simulink model "velocityInRadiusOut"  (R2019a)
settings: Solver=VariableStepAuto  StartTime=0  StopTime=init.maxV  MaxStep=1e-3  RelTol=1e-3
undefined symbols (not defined in the file or in its folder): init
libraries: simulink x1
settings Model: Creator=fried  LastModifiedBy=fried

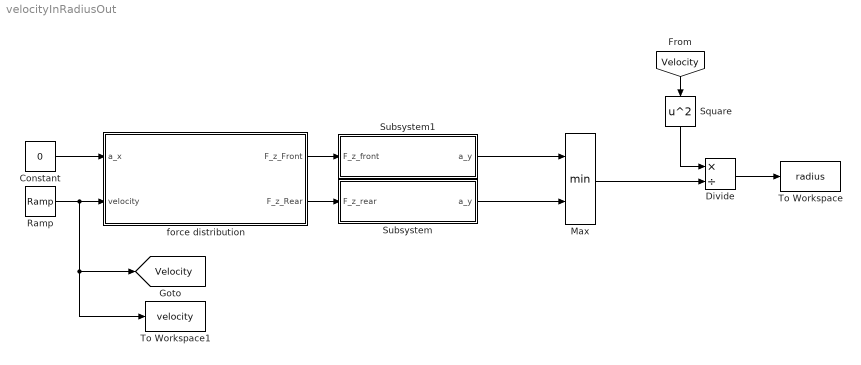
== system velocityInRadiusOut ==
  Constant : Constant  Value=0
  Divide : Product  Inputs=*/
  Max : MinMax  Inputs=2
  Ramp : simulink/Sources/Ramp  slope=1  start=0  InitialOutput=0
  Square : Math  Operator=square  SaturateOnIntegerOverflow=on
  Subsystem : Subsystem
  Subsystem1 : Subsystem
  To Workspace : ToWorkspace  VariableName=radius  SampleTime=-1
  To Workspace1 : ToWorkspace  VariableName=velocity  SampleTime=-1
  force distribution : Subsystem
  tag scope: Velocity=global
  wires:
  Ramp/1 -> To Workspace1/1, [Velocity], force distribution/2("velocity ")
  force distribution/2("F_z_Rear ") -> Subsystem/1("F_z_rear ")
  force distribution/1(F_z_Front) -> Subsystem1/1(F_z_front)
  Subsystem1/1(a_y) -> Max/1
  [Velocity] -> Square/1
  Square/1 -> Divide/1
  Max/1 -> Divide/2
  Divide/1 -> To Workspace/1
  Subsystem/1(a_y) -> Max/2
  Constant/1 -> force distribution/1("a_x ")

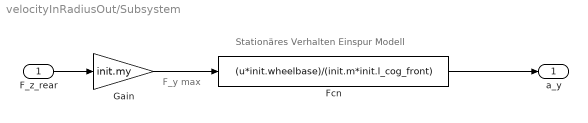
== system velocityInRadiusOut/Subsystem ==
  note: Stationäres Verhalten Einspur Modell
  note: F_y max
  "F_z_rear " : Inport
  Fcn : Fcn  Expr=(u*init.wheelbase)/(init.m*init.l_cog_front)
  Gain : Gain  Gain=init.my
  a_y : Outport
  wires:
  Gain/1 -> Fcn/1
  "F_z_rear "/1 -> Gain/1
  Fcn/1 -> a_y/1

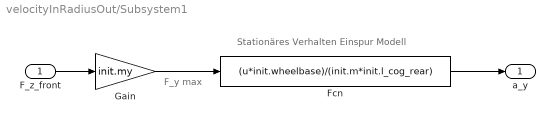
== system velocityInRadiusOut/Subsystem1 ==
  note: F_y max
  note: Stationäres Verhalten Einspur Modell
  F_z_front : Inport
  Fcn : Fcn  Expr=(u*init.wheelbase)/(init.m*init.l_cog_rear)
  Gain : Gain  Gain=init.my
  a_y : Outport
  wires:
  Fcn/1 -> a_y/1
  F_z_front/1 -> Gain/1
  Gain/1 -> Fcn/1

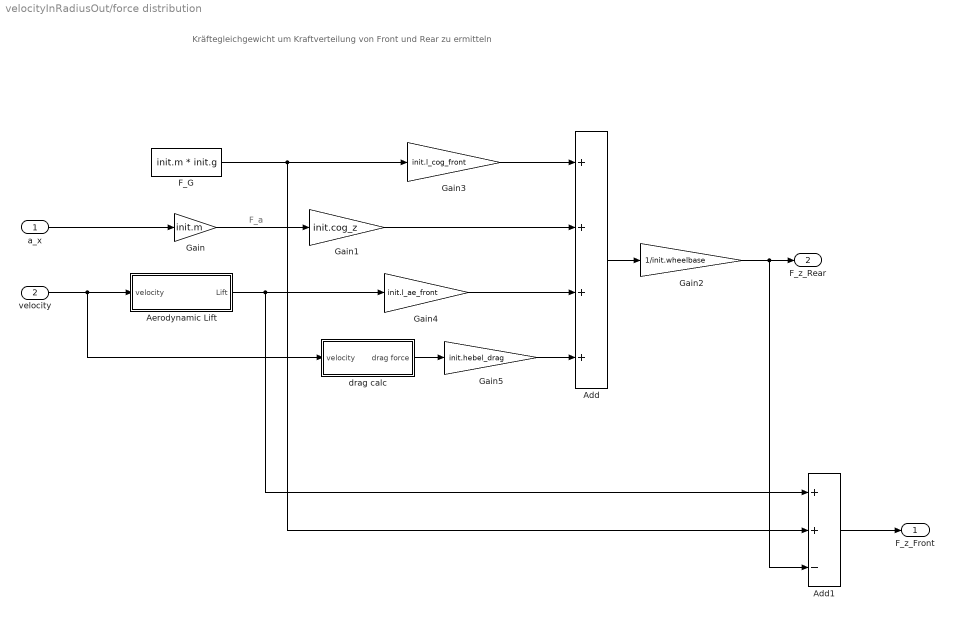
== system velocityInRadiusOut/force distribution ==
  note: Kräftegleichgewicht um Kraftverteilung von Front und Rear zu ermitteln
  note: F_a
  "a_x " : Inport
  "velocity " : Inport  Port=2
  Add : Sum  Inputs=++++
  Add1 : Sum  Inputs=++-
  Aerodynamic Lift : Subsystem
  "F_G " : Constant  Value=init.m * init.g
  Gain : Gain  Gain=init.m
  Gain1 : Gain  Gain=init.cog_z
  Gain2 : Gain  Gain=1/init.wheelbase
  Gain3 : Gain  Gain=init.l_cog_front
  Gain4 : Gain  Gain=init.l_ae_front
  Gain5 : Gain  Gain=init.hebel_drag
  drag calc : Subsystem
  F_z_Front : Outport
  "F_z_Rear " : Outport  Port=2
  wires:
  "a_x "/1 -> Gain/1
  "F_G "/1 -> Add1/2, Gain3/1
  Gain3/1 -> Add/1
  Gain/1 -> Gain1/1
  "velocity "/1 -> drag calc/1(velocity), Aerodynamic Lift/1(velocity)
  Aerodynamic Lift/1(Lift) -> Gain4/1, Add1/1
  Gain1/1 -> Add/2
  Gain4/1 -> Add/3
  Add/1 -> Gain2/1
  Gain2/1 -> Add1/3, "F_z_Rear "/1
  Add1/1 -> F_z_Front/1
  Gain5/1 -> Add/4
  drag calc/1("drag force ") -> Gain5/1

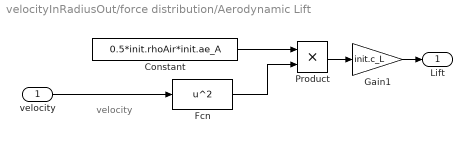
== system velocityInRadiusOut/force distribution/Aerodynamic Lift ==
  note: velocity
  velocity : Inport
  Constant : Constant  Value=0.5*init.rhoAir*init.ae_A
  Fcn : Fcn  Expr=u^2
  Gain1 : Gain  Gain=init.c_L
  Product : Product
  Lift : Outport
  wires:
  Fcn/1 -> Product/2
  velocity/1 -> Fcn/1
  Constant/1 -> Product/1
  Product/1 -> Gain1/1
  Gain1/1 -> Lift/1

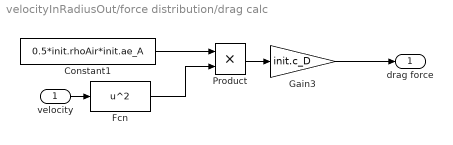
== system velocityInRadiusOut/force distribution/drag calc ==
  velocity : Inport
  Constant1 : Constant  Value=0.5*init.rhoAir*init.ae_A
  Fcn : Fcn  Expr=u^2
  Gain3 : Gain  Gain=init.c_D
  Product : Product
  "drag force " : Outport
  wires:
  Constant1/1 -> Product/1
  velocity/1 -> Fcn/1
  Fcn/1 -> Product/2
  Product/1 -> Gain3/1
  Gain3/1 -> "drag force "/1
